simulink library "inp"  (R2021b)
settings: Solver=VariableStepAuto  StartTime=0.0  StopTime=10.0  RelTol=1e-3
undefined symbols (not defined in the file): C_TASK_5MS_S, FALSE, KINP_AcoreReadyToSlp_flg_ovrdflg, KINP_AcoreReadyToSlp_flg_ovrdval, KINP_AllowMovThd_OTA_enum_ovrdflg, KINP_AllowMovThd_OTA_enum_ovrdval, KINP_APSAngleTarget_Deg_ovrdflg, KINP_APSAngleTarget_Deg_ovrdval, KINP_APSDecReq_mps2_ovrdflg, KINP_APSDecReq_mps2_ovrdval, KINP_APSDecReqA_flg_ovrdflg, KINP_APSDecReqA_flg_ovrdval, KINP_APSDFLL_cm_ovrdflg, KINP_APSDFLL_cm_ovrdval, KINP_APSDFLR_cm_ovrdflg, KINP_APSDFLR_cm_ovrdval, KINP_APSDRLL_cm_ovrdflg, KINP_APSDRLL_cm_ovrdval, KINP_APSDRLR_cm_ovrdflg, KINP_APSDRLR_cm_ovrdval, KINP_APSExitCondition_enum_ovrdflg, KINP_APSExitCondition_enum_ovrdval, KINP_APSHWVer_enum_ovrdflg, KINP_APSHWVer_enum_ovrdval, KINP_APSProgressPCT_pct_ovrdflg, KINP_APSProgressPCT_pct_ovrdval, KINP_APSPwrReq_enum_ovrdflg, KINP_APSPwrReq_enum_ovrdval, KINP_APSReq_enum_ovrdflg, KINP_APSReq_enum_ovrdval, KINP_APSRQDisplay_enum_ovrdflg, KINP_APSRQDisplay_enum_ovrdval, KINP_APSRqEPASCtrl_flg_ovrdflg, KINP_APSRqEPASCtrl_flg_ovrdval, KINP_APSShiftPosnReq_enum_ovrdval, KINP_APSShiftPosnReq_enum_ovrflg, KINP_APSSpeedCMD_kph_ovrdval, KINP_APSSpeedCMD_kph_ovrflg, KINP_APSStaSystem_enum_ovrdflg, KINP_APSStaSystem_enum_ovrdval, KINP_APSSWVer_enum_ovrdflg, KINP_APSSWVer_enum_ovrdval, KINP_APSVMCReqA_flg_ovrdval, KINP_APSVMCReqA_flg_ovrflg, KINP_APSVRqEPASCtrl_flg_ovrdflg, KINP_APSVRqEPASCtrl_flg_ovrdval, KINP_AuxBattVolmV_mV_ovrdflg, KINP_AuxBattVolmV_mV_ovrdval, KINP_CAASSta_enum_ovrdflg, KINP_CAASSta_enum_ovrdval, KINP_CAASVMCReqA_flg_ovrdval, KINP_CAASVMCReqA_flg_ovrflg, KINP_CAN1BusOff_flg_ovrdflg, KINP_CAN1BusOff_flg_ovrdval, KINP_CAN2BusOff_flg_ovrdflg, KINP_CAN2BusOff_flg_ovrdval, KINP_CAN3BusOff_flg_ovrdflg, KINP_CAN3BusOff_flg_ovrdval, KINP_CAN4BusOff_flg_ovrdflg, KINP_CAN4BusOff_flg_ovrdval ... (+152)
libraries: FVT_lib x1035, hcu_lib x1
(part 31 of 33)

== system inp/INP/CAN5/SignalCheck/TBOX3 ==
  BHAL_outputs : Inport
  inp_CanValid_bus : Inport  Port=2
  ChargePercentSet : FVT_lib/inp/can_signal_template  SystemSampleTime=-1  VariantActivationTime=update diagram  Latency=0  AutoFrameSizeCalculation=off
      link override defval: Value=KINP_ChargePercentSet_pct_defval
      link override ovrdflg: Value=KINP_ChargePercentSet_pct_ovrdflg
      link override ovrdval: Value=KINP_ChargePercentSet_pct_ovrdval
  ReserveChargeOFFDay : FVT_lib/inp/can_signal_template  SystemSampleTime=-1  VariantActivationTime=update diagram  Latency=0  AutoFrameSizeCalculation=off
      link override defval: Value=KINP_ReserveChargeOFFDay_DAY_defval
      link override ovrdflg: Value=KINP_ReserveChargeOFFDay_DAY_ovrdflg
      link override ovrdval: Value=KINP_ReserveChargeOFFDay_DAY_ovrdval
  ReserveChargeOFFHour : FVT_lib/inp/can_signal_template  SystemSampleTime=-1  VariantActivationTime=update diagram  Latency=0  AutoFrameSizeCalculation=off
      link override defval: Value=KINP_ReserveChargeOFFHour_hr_defval
      link override ovrdflg: Value=KINP_ReserveChargeOFFHour_hr_ovrdflg
      link override ovrdval: Value=KINP_ReserveChargeOFFHour_hr_ovrdval
  ReserveChargeOFFMinute : FVT_lib/inp/can_signal_template  SystemSampleTime=-1  VariantActivationTime=update diagram  Latency=0  AutoFrameSizeCalculation=off
      link override defval: Value=KINP_ReserveChargeOFFMinute_min_defval
      link override ovrdflg: Value=KINP_ReserveChargeOFFMinute_min_ovrdflg
      link override ovrdval: Value=KINP_ReserveChargeOFFMinute_min_ovrdval
  ReserveChargeOFFMonth : FVT_lib/inp/can_signal_template  SystemSampleTime=-1  VariantActivationTime=update diagram  Latency=0  AutoFrameSizeCalculation=off
      link override defval: Value=KINP_ReserveChargeOFFMonth_MONTH_defval
      link override ovrdflg: Value=KINP_ReserveChargeOFFMonth_MONTH_ovrdflg
      link override ovrdval: Value=KINP_ReserveChargeOFFMonth_MONTH_ovrdval
  ReserveChargeOFFYear : FVT_lib/inp/can_signal_template  SystemSampleTime=-1  VariantActivationTime=update diagram  Latency=0  AutoFrameSizeCalculation=off
      link override defval: Value=KINP_ReserveChargeOFFYear_YEAR_defval
      link override ovrdflg: Value=KINP_ReserveChargeOFFYear_YEAR_ovrdflg
      link override ovrdval: Value=KINP_ReserveChargeOFFYear_YEAR_ovrdval
  ReserveChargeOnDay : FVT_lib/inp/can_signal_template  SystemSampleTime=-1  VariantActivationTime=update diagram  Latency=0  AutoFrameSizeCalculation=off
      link override defval: Value=KINP_ReserveChargeOnDay_DAY_defval
      link override ovrdflg: Value=KINP_ReserveChargeOnDay_DAY_ovrdflg
      link override ovrdval: Value=KINP_ReserveChargeOnDay_DAY_ovrdval
  ReserveChargeOnHour : FVT_lib/inp/can_signal_template  SystemSampleTime=-1  VariantActivationTime=update diagram  Latency=0  AutoFrameSizeCalculation=off
      link override defval: Value=KINP_ReserveChargeOnHour_hr_defval
      link override ovrdflg: Value=KINP_ReserveChargeOnHour_hr_ovrdflg
      link override ovrdval: Value=KINP_ReserveChargeOnHour_hr_ovrdval
  ReserveChargeOnMinute : FVT_lib/inp/can_signal_template  SystemSampleTime=-1  VariantActivationTime=update diagram  Latency=0  AutoFrameSizeCalculation=off
      link override defval: Value=KINP_ReserveChargeOnMinute_min_defval
      link override ovrdflg: Value=KINP_ReserveChargeOnMinute_min_ovrdflg
      link override ovrdval: Value=KINP_ReserveChargeOnMinute_min_ovrdval
  ReserveChargeOnMonth : FVT_lib/inp/can_signal_template  SystemSampleTime=-1  VariantActivationTime=update diagram  Latency=0  AutoFrameSizeCalculation=off
      link override defval: Value=KINP_ReserveChargeOnMonth_MONTH_defval
      link override ovrdflg: Value=KINP_ReserveChargeOnMonth_MONTH_ovrdflg
      link override ovrdval: Value=KINP_ReserveChargeOnMonth_MONTH_ovrdval
  ReserveChargeOnYear : FVT_lib/inp/can_signal_template  SystemSampleTime=-1  VariantActivationTime=update diagram  Latency=0  AutoFrameSizeCalculation=off
      link override defval: Value=KINP_ReserveChargeOnYear_YEAR_defval
      link override ovrdflg: Value=KINP_ReserveChargeOnYear_YEAR_ovrdflg
      link override ovrdval: Value=KINP_ReserveChargeOnYear_YEAR_ovrdval
  TBOXHWVER : FVT_lib/inp/can_signal_template  SystemSampleTime=-1  VariantActivationTime=update diagram  Latency=0  AutoFrameSizeCalculation=off
      link override defval: Value=KINP_TBOXHWVER_enum_defval
      link override ovrdflg: Value=KINP_TBOXHWVER_enum_ovrdflg
      link override ovrdval: Value=KINP_TBOXHWVER_enum_ovrdval
  TBOXSWVER : FVT_lib/inp/can_signal_template  SystemSampleTime=-1  VariantActivationTime=update diagram  Latency=0  AutoFrameSizeCalculation=off
      link override defval: Value=KINP_TBOXSWVER_enum_defval
      link override ovrdflg: Value=KINP_TBOXSWVER_enum_ovrdflg
      link override ovrdval: Value=KINP_TBOXSWVER_enum_ovrdval
  Terminator_{1..13} (13 alike) : Terminator
  True_VHAL_ChargePercentSet_pct : Constant  Value=TRUE  OutDataTypeStr=boolean
  True_VHAL_ReserveChargeOFFDay_DAY : Constant  Value=TRUE  OutDataTypeStr=boolean
  True_VHAL_ReserveChargeOFFHour_hr : Constant  Value=TRUE  OutDataTypeStr=boolean
  True_VHAL_ReserveChargeOFFMinute_min : Constant  Value=TRUE  OutDataTypeStr=boolean
  True_VHAL_ReserveChargeOFFMonth_MONTH : Constant  Value=TRUE  OutDataTypeStr=boolean
  True_VHAL_ReserveChargeOFFYear_YEAR : Constant  Value=TRUE  OutDataTypeStr=boolean
  True_VHAL_ReserveChargeOnDay_DAY : Constant  Value=TRUE  OutDataTypeStr=boolean
  True_VHAL_ReserveChargeOnHour_hr : Constant  Value=TRUE  OutDataTypeStr=boolean
  True_VHAL_ReserveChargeOnMinute_min : Constant  Value=TRUE  OutDataTypeStr=boolean
  True_VHAL_ReserveChargeOnMonth_MONTH : Constant  Value=TRUE  OutDataTypeStr=boolean
  True_VHAL_ReserveChargeOnYear_YEAR : Constant  Value=TRUE  OutDataTypeStr=boolean
  True_VHAL_TBOXHWVER_enum : Constant  Value=TRUE  OutDataTypeStr=boolean
  True_VHAL_TBOXSWVER_enum : Constant  Value=TRUE  OutDataTypeStr=boolean
  slr1_{1..13} (13 alike) : BusSelector  OutputSignals=VINP_CANMsgValidTBOX3_flg
  slr_VHAL_ChargePercentSet_pct : BusSelector  OutputSignals=VHAL_ChargePercentSet_pct
  slr_VHAL_ReserveChargeOFFDay_DAY : BusSelector  OutputSignals=VHAL_ReserveChargeOFFDay_DAY
  slr_VHAL_ReserveChargeOFFHour_hr : BusSelector  OutputSignals=VHAL_ReserveChargeOFFHour_hr
  slr_VHAL_ReserveChargeOFFMinute_min : BusSelector  OutputSignals=VHAL_ReserveChargeOFFMinute_min
  slr_VHAL_ReserveChargeOFFMonth_MONTH : BusSelector  OutputSignals=VHAL_ReserveChargeOFFMonth_MONTH
  slr_VHAL_ReserveChargeOFFYear_YEAR : BusSelector  OutputSignals=VHAL_ReserveChargeOFFYear_YEAR
  slr_VHAL_ReserveChargeOnDay_DAY : BusSelector  OutputSignals=VHAL_ReserveChargeOnDay_DAY
  slr_VHAL_ReserveChargeOnHour_hr : BusSelector  OutputSignals=VHAL_ReserveChargeOnHour_hr
  slr_VHAL_ReserveChargeOnMinute_min : BusSelector  OutputSignals=VHAL_ReserveChargeOnMinute_min
  slr_VHAL_ReserveChargeOnMonth_MONTH : BusSelector  OutputSignals=VHAL_ReserveChargeOnMonth_MONTH
  slr_VHAL_ReserveChargeOnYear_YEAR : BusSelector  OutputSignals=VHAL_ReserveChargeOnYear_YEAR
  slr_VHAL_TBOXHWVER_enum : BusSelector  OutputSignals=VHAL_TBOXHWVER_enum
  slr_VHAL_TBOXSWVER_enum : BusSelector  OutputSignals=VHAL_TBOXSWVER_enum
  VINP_ChargePercentSet_pct : Outport
  VINP_ReserveChargeOFFDay_DAY : Outport  Port=2
  VINP_ReserveChargeOFFHour_hr : Outport  Port=3
  VINP_ReserveChargeOFFMinute_min : Outport  Port=4
  VINP_ReserveChargeOFFMonth_MONTH : Outport  Port=5
  VINP_ReserveChargeOFFYear_YEAR : Outport  Port=6
  VINP_ReserveChargeOnDay_DAY : Outport  Port=7
  VINP_ReserveChargeOnHour_hr : Outport  Port=8
  VINP_ReserveChargeOnMinute_min : Outport  Port=9
  VINP_ReserveChargeOnMonth_MONTH : Outport  Port=10
  VINP_ReserveChargeOnYear_YEAR : Outport  Port=11
  VINP_TBOXHWVER_enum : Outport  Port=12
  VINP_TBOXSWVER_enum : Outport  Port=13
  wires:
  BHAL_outputs/1 -> [BHAL_outputs]
  inp_CanValid_bus/1 -> [inp_CanValid_bus]
  [BHAL_outputs] -> slr_VHAL_ChargePercentSet_pct/1
  slr_VHAL_ChargePercentSet_pct/1 -> ChargePercentSet/1  "<VHAL_ChargePercentSet_pct>"
  True_VHAL_ChargePercentSet_pct/1 -> ChargePercentSet/2
  [inp_CanValid_bus] -> slr1_1/1
  slr1_1/1 -> ChargePercentSet/3  "<VINP_CANMsgValidTBOX3_flg>"
  ChargePercentSet/1 -> VINP_ChargePercentSet_pct/1  "VINP_ChargePercentSet_pct"
  ChargePercentSet/2 -> Terminator_1/1
  [BHAL_outputs] -> slr_VHAL_ReserveChargeOFFDay_DAY/1
  slr_VHAL_ReserveChargeOFFDay_DAY/1 -> ReserveChargeOFFDay/1  "<VHAL_ReserveChargeOFFDay_DAY>"
  True_VHAL_ReserveChargeOFFDay_DAY/1 -> ReserveChargeOFFDay/2
  [inp_CanValid_bus] -> slr1_2/1
  slr1_2/1 -> ReserveChargeOFFDay/3  "<VINP_CANMsgValidTBOX3_flg>"
  ReserveChargeOFFDay/1 -> VINP_ReserveChargeOFFDay_DAY/1  "VINP_ReserveChargeOFFDay_DAY"
  ReserveChargeOFFDay/2 -> Terminator_2/1
  [BHAL_outputs] -> slr_VHAL_ReserveChargeOFFHour_hr/1
  slr_VHAL_ReserveChargeOFFHour_hr/1 -> ReserveChargeOFFHour/1  "<VHAL_ReserveChargeOFFHour_hr>"
  True_VHAL_ReserveChargeOFFHour_hr/1 -> ReserveChargeOFFHour/2
  [inp_CanValid_bus] -> slr1_3/1
  slr1_3/1 -> ReserveChargeOFFHour/3  "<VINP_CANMsgValidTBOX3_flg>"
  ReserveChargeOFFHour/1 -> VINP_ReserveChargeOFFHour_hr/1  "VINP_ReserveChargeOFFHour_hr"
  ReserveChargeOFFHour/2 -> Terminator_3/1
  [BHAL_outputs] -> slr_VHAL_ReserveChargeOFFMinute_min/1
  slr_VHAL_ReserveChargeOFFMinute_min/1 -> ReserveChargeOFFMinute/1  "<VHAL_ReserveChargeOFFMinute_min>"
  True_VHAL_ReserveChargeOFFMinute_min/1 -> ReserveChargeOFFMinute/2
  [inp_CanValid_bus] -> slr1_4/1
  slr1_4/1 -> ReserveChargeOFFMinute/3  "<VINP_CANMsgValidTBOX3_flg>"
  ReserveChargeOFFMinute/1 -> VINP_ReserveChargeOFFMinute_min/1  "VINP_ReserveChargeOFFMinute_min"
  ReserveChargeOFFMinute/2 -> Terminator_4/1
  [BHAL_outputs] -> slr_VHAL_ReserveChargeOFFMonth_MONTH/1
  slr_VHAL_ReserveChargeOFFMonth_MONTH/1 -> ReserveChargeOFFMonth/1  "<VHAL_ReserveChargeOFFMonth_MONTH>"
  True_VHAL_ReserveChargeOFFMonth_MONTH/1 -> ReserveChargeOFFMonth/2
  [inp_CanValid_bus] -> slr1_5/1
  slr1_5/1 -> ReserveChargeOFFMonth/3  "<VINP_CANMsgValidTBOX3_flg>"
  ReserveChargeOFFMonth/1 -> VINP_ReserveChargeOFFMonth_MONTH/1  "VINP_ReserveChargeOFFMonth_MONTH"
  ReserveChargeOFFMonth/2 -> Terminator_5/1
  [BHAL_outputs] -> slr_VHAL_ReserveChargeOFFYear_YEAR/1
  slr_VHAL_ReserveChargeOFFYear_YEAR/1 -> ReserveChargeOFFYear/1  "<VHAL_ReserveChargeOFFYear_YEAR>"
  True_VHAL_ReserveChargeOFFYear_YEAR/1 -> ReserveChargeOFFYear/2
  [inp_CanValid_bus] -> slr1_6/1
  slr1_6/1 -> ReserveChargeOFFYear/3  "<VINP_CANMsgValidTBOX3_flg>"
  ReserveChargeOFFYear/1 -> VINP_ReserveChargeOFFYear_YEAR/1  "VINP_ReserveChargeOFFYear_YEAR"
  ReserveChargeOFFYear/2 -> Terminator_6/1
  [BHAL_outputs] -> slr_VHAL_ReserveChargeOnDay_DAY/1
  slr_VHAL_ReserveChargeOnDay_DAY/1 -> ReserveChargeOnDay/1  "<VHAL_ReserveChargeOnDay_DAY>"
  True_VHAL_ReserveChargeOnDay_DAY/1 -> ReserveChargeOnDay/2
  [inp_CanValid_bus] -> slr1_7/1
  slr1_7/1 -> ReserveChargeOnDay/3  "<VINP_CANMsgValidTBOX3_flg>"
  ReserveChargeOnDay/1 -> VINP_ReserveChargeOnDay_DAY/1  "VINP_ReserveChargeOnDay_DAY"
  ReserveChargeOnDay/2 -> Terminator_7/1
  [BHAL_outputs] -> slr_VHAL_ReserveChargeOnHour_hr/1
  slr_VHAL_ReserveChargeOnHour_hr/1 -> ReserveChargeOnHour/1  "<VHAL_ReserveChargeOnHour_hr>"
  True_VHAL_ReserveChargeOnHour_hr/1 -> ReserveChargeOnHour/2
  [inp_CanValid_bus] -> slr1_8/1
  slr1_8/1 -> ReserveChargeOnHour/3  "<VINP_CANMsgValidTBOX3_flg>"
  ReserveChargeOnHour/1 -> VINP_ReserveChargeOnHour_hr/1  "VINP_ReserveChargeOnHour_hr"
  ReserveChargeOnHour/2 -> Terminator_8/1
  [BHAL_outputs] -> slr_VHAL_ReserveChargeOnMinute_min/1
  slr_VHAL_ReserveChargeOnMinute_min/1 -> ReserveChargeOnMinute/1  "<VHAL_ReserveChargeOnMinute_min>"
  True_VHAL_ReserveChargeOnMinute_min/1 -> ReserveChargeOnMinute/2
  [inp_CanValid_bus] -> slr1_9/1
  slr1_9/1 -> ReserveChargeOnMinute/3  "<VINP_CANMsgValidTBOX3_flg>"
  ReserveChargeOnMinute/1 -> VINP_ReserveChargeOnMinute_min/1  "VINP_ReserveChargeOnMinute_min"
  ReserveChargeOnMinute/2 -> Terminator_9/1
  [BHAL_outputs] -> slr_VHAL_ReserveChargeOnMonth_MONTH/1
  slr_VHAL_ReserveChargeOnMonth_MONTH/1 -> ReserveChargeOnMonth/1  "<VHAL_ReserveChargeOnMonth_MONTH>"
  True_VHAL_ReserveChargeOnMonth_MONTH/1 -> ReserveChargeOnMonth/2
  [inp_CanValid_bus] -> slr1_10/1
  slr1_10/1 -> ReserveChargeOnMonth/3  "<VINP_CANMsgValidTBOX3_flg>"
  ReserveChargeOnMonth/1 -> VINP_ReserveChargeOnMonth_MONTH/1  "VINP_ReserveChargeOnMonth_MONTH"
  ReserveChargeOnMonth/2 -> Terminator_10/1
  [BHAL_outputs] -> slr_VHAL_ReserveChargeOnYear_YEAR/1
  slr_VHAL_ReserveChargeOnYear_YEAR/1 -> ReserveChargeOnYear/1  "<VHAL_ReserveChargeOnYear_YEAR>"
  True_VHAL_ReserveChargeOnYear_YEAR/1 -> ReserveChargeOnYear/2
  [inp_CanValid_bus] -> slr1_11/1
  slr1_11/1 -> ReserveChargeOnYear/3  "<VINP_CANMsgValidTBOX3_flg>"
  ReserveChargeOnYear/1 -> VINP_ReserveChargeOnYear_YEAR/1  "VINP_ReserveChargeOnYear_YEAR"
  ReserveChargeOnYear/2 -> Terminator_11/1
  [BHAL_outputs] -> slr_VHAL_TBOXHWVER_enum/1
  slr_VHAL_TBOXHWVER_enum/1 -> TBOXHWVER/1  "<VHAL_TBOXHWVER_enum>"
  True_VHAL_TBOXHWVER_enum/1 -> TBOXHWVER/2
  [inp_CanValid_bus] -> slr1_12/1
  slr1_12/1 -> TBOXHWVER/3  "<VINP_CANMsgValidTBOX3_flg>"
  TBOXHWVER/1 -> VINP_TBOXHWVER_enum/1  "VINP_TBOXHWVER_enum"
  TBOXHWVER/2 -> Terminator_12/1
  [BHAL_outputs] -> slr_VHAL_TBOXSWVER_enum/1
  slr_VHAL_TBOXSWVER_enum/1 -> TBOXSWVER/1  "<VHAL_TBOXSWVER_enum>"
  True_VHAL_TBOXSWVER_enum/1 -> TBOXSWVER/2
  [inp_CanValid_bus] -> slr1_13/1
  slr1_13/1 -> TBOXSWVER/3  "<VINP_CANMsgValidTBOX3_flg>"
  TBOXSWVER/1 -> VINP_TBOXSWVER_enum/1  "VINP_TBOXSWVER_enum"
  TBOXSWVER/2 -> Terminator_13/1
